simulink model "propeller_openloop_control"  (R2021b)
settings: Solver=VariableStepAuto  StartTime=0.0  StopTime=1  RelTol=1e-3
undefined symbols (not defined in the file or in its folder): k
settings Model: Creator=cirie  LastModifiedBy=cirie

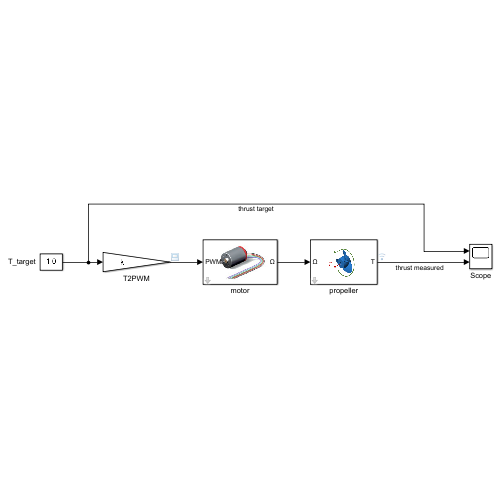
[thumbnail: Simulink's stored preview of the top-level diagram]
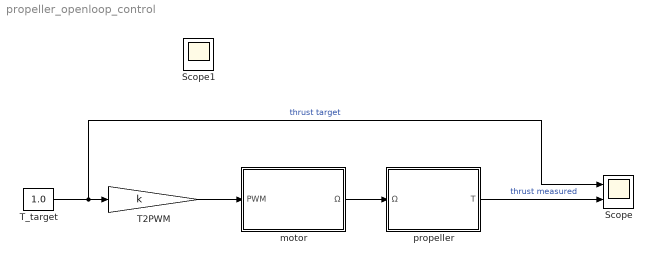
== system propeller_openloop_control ==
  Scope : Scope  NumInputPorts=2
  T2PWM : Gain  Gain=k
  T_target : Constant  Value=1.0  SampleTime=0.1
  motor : Subsystem  mask(DC Motor){J=1e-4, km=0.1, R=1, Vmax=7.2}
      mask prompts: J "Inertia, J [kgm^2]"; km "Motor constant, km [V*s/rad]"; R "Resistance, R [Ohm]"; Vmax "Maximum Voltage, Vmax [V]"
      mask help:
      | Circuit Dynamics:   PWM*Vmax == I*R + km*Ω
      | Rotor Dynamics:     J*dΩ/dt == km*I
      mask Display: image('$imagefile'); % Use "Edit Image" on toolstrip to change.
  propeller : Subsystem  mask(Propeller Model){D=0.1, kt=0.01, rho=1000}
      mask prompts: D "Propeller Diameter [m]"; kt "Thrust Coefficient"; rho "Fluid density [kg/m^3]"
      mask help: Propeller Dynamics: T = kt*rho*omega^2*D^4
      mask Display: image('$imagefile'); % Use "Edit Image" on toolstrip to change.
  Scope1 : Scope
  wires:
  propeller/1(T) -> Scope/2  "thrust measured"
  T_target/1 -> Scope/1, T2PWM/1  "thrust target"
  motor/1(Ω) -> propeller/1(Ω)
  T2PWM/1 -> motor/1(PWM)

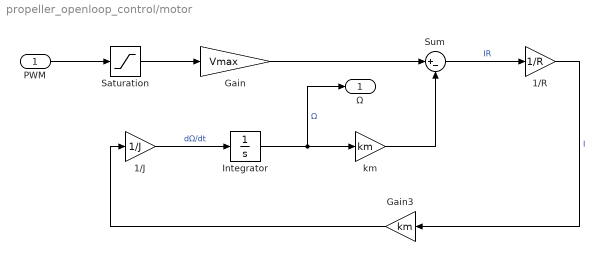
== system propeller_openloop_control/motor ==
  PWM : Inport
  1/J : Gain  Gain=1/J
  1/R : Gain  Gain=1/R
  Gain : Gain  Gain=Vmax
  Gain3 : Gain  Gain=km
  Integrator : Integrator
  Saturation : Saturate  UpperLimit=1  LowerLimit=-1
  Sum : Sum  Inputs=|+-
  km : Gain  Gain=km
  Ω : Outport
  wires:
  1/J/1 -> Integrator/1  "dΩ/dt"
  Sum/1 -> 1/R/1  "IR"
  Integrator/1 -> Ω/1, km/1  "Ω"
  Gain3/1 -> 1/J/1
  km/1 -> Sum/2
  1/R/1 -> Gain3/1  "I"
  PWM/1 -> Saturation/1
  Gain/1 -> Sum/1
  Saturation/1 -> Gain/1

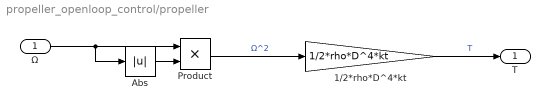
== system propeller_openloop_control/propeller ==
  Ω : Inport
  1/2*rho*D^4*kt : Gain  Gain=1/2*rho*D^4*kt
  Abs : Abs
  Product : Product
  T : Outport
  wires:
  1/2*rho*D^4*kt/1 -> T/1  "T"
  Product/1 -> 1/2*rho*D^4*kt/1  "Ω^2"
  Ω/1 -> Abs/1, Product/1
  Abs/1 -> Product/2
